simulink model "permisosolo"  (R2020b)
settings: Solver=VariableStepAuto  StartTime=0.0  StopTime=10.0  RelTol=1e-3
settings Model: Creator=cacha  LastModifiedBy=cacha

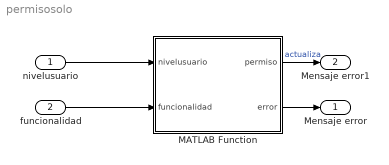
== system permisosolo ==
  nivelusuario : Inport
  funcionalidad : Inport  Port=2
  MATLAB Function : MATLAB Function  TreatAsAtomicUnit=on
  Mensaje error : Outport  SignalName=H  OutMin=0  OutMax=1  OutDataTypeStr=double  PortDimensions=1
      settings: MustResolveToSignalObject=on
  Mensaje error1 : Outport  Port=2  SignalName=H  OutMin=0  OutMax=1  OutDataTypeStr=double  PortDimensions=1
      settings: MustResolveToSignalObject=on
  wires:
  funcionalidad/1 -> MATLAB Function/2(funcionalidad)
  nivelusuario/1 -> MATLAB Function/1(nivelusuario)
  MATLAB Function/2(error) -> Mensaje error/1
  MATLAB Function/1(permiso) -> Mensaje error1/1  "actualiza"

== matlab function permisosolo/MATLAB Function ==
  data: nivelusuario input; permiso output; funcionalidad input; error output
function [permiso,error] = fcn(nivelusuario, funcionalidad)

if nivelusuario == 1 && (funcionalidad == 1 || funcionalidad == 2 || funcionalidad ==3)
    permiso = 1;
    error = 0;   
elseif nivelusuario == 2 && (funcionalidad == 2 || funcionalidad ==3)
    permiso = 1;
    error = 0;    
elseif nivelusuario ==3 && funcionalidad == 3
    permiso = 1;
    error = 0;

else 
    permiso = 0;
    error = 0;
end

if nivelusuario > funcionalidad 
    error = 1;
end

end
